simulink model "inverter"  (R2020a)
settings: Solver=VariableStepAuto  StartTime=0.0  StopTime=0.5  RelTol=1e-3
libraries: powerlib x15
settings Model: Creator=chrishao  LastModifiedBy=chrishao

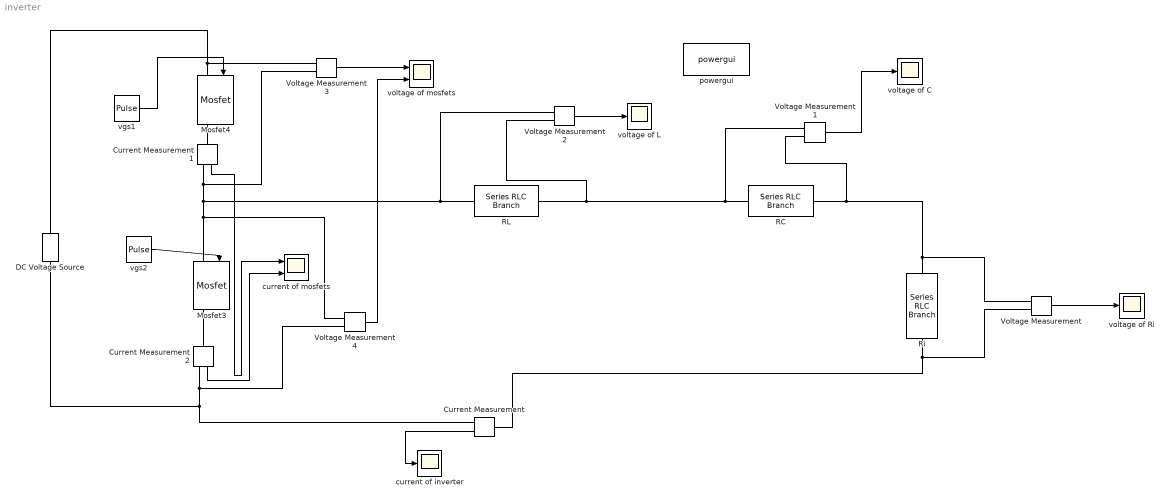
== system inverter ==
  Current Measurement : powerlib/Measurements/Current Measurement  PhasorSimulation=off  OutputType=Complex  PSBequivalent=0
  Current Measurement1 : powerlib/Measurements/Current Measurement  PhasorSimulation=off  OutputType=Complex  PSBequivalent=0
  Current Measurement2 : powerlib/Measurements/Current Measurement  PhasorSimulation=off  OutputType=Complex  PSBequivalent=0
  DC Voltage Source : powerlib/Electrical Sources/DC Voltage Source  Amplitude=180  Measurements=None
  Mosfet3 : powerlib/Power Electronics/Mosfet  Ron=1.4243  Lon=0  Rd=0.01  Vfd=0  IC=0  Rs=1e5  Cs=inf  Measurements=on
  Mosfet4 : powerlib/Power Electronics/Mosfet  Ron=1.4243  Lon=0  Rd=0.01  Vfd=0  IC=0  Rs=1e5  Cs=inf  Measurements=on
  RC : powerlib/Elements/Series RLC Branch  LConnTagsString=__new0  RConnTagsString=__new0  BranchType=RC  Resistance=0.7957  Inductance=675.2e-3  SetiL0=off  InitialCurrent=0  Capacitance=937.86e-12  Setx0=off  InitialVoltage=0  Measurements=None
  RL : powerlib/Elements/Series RLC Branch  LConnTagsString=__new0  RConnTagsString=__new0  BranchType=RL  Resistance=3.5090  Inductance=675.2e-6  SetiL0=off  InitialCurrent=0  Capacitance=1e-6  Setx0=off  InitialVoltage=0  Measurements=None
  Ri : powerlib/Elements/Series RLC Branch  LConnTagsString=__new0  RConnTagsString=__new0  BranchType=R  Resistance=137.4937  Inductance=675.2e-3  SetiL0=off  InitialCurrent=0  Capacitance=10e-9  Setx0=off  InitialVoltage=0  Measurements=None
  Voltage Measurement{,1..4} (5 alike) : powerlib/Measurements/Voltage Measurement  PhasorSimulation=off  OutputType=Complex  PSBequivalent=0
  current of inverter : Scope
  current of mosfets : Scope  NumInputPorts=2
  powergui : powerlib/powergui  Priority=1  SimulationMode=Continuous  SampleTime=50e-6  frequency=60  Iterations=50  frequencyindice=0  Pbase=100e6  ErrMax=1e-4  UnitsV=kV  UnitsW=MW  buscounter=0  FunctionMessages=off  echomessages=off  EnableUseOfTLC=off  CurrentSourceSwitches=off  DisableSnubberDevices=off  DisableRonSwitches=off  DisableVfSwitches=off  DisplayEquations=off  AutomaticDiscreteSolvers=off  SolverType=Tustin/Backward Euler (TBE)  Interpol=off  ExternalGateDelay=off  methode=off  Ts=100  x0status=blocks  SPID=on  SwTol=0  HookPort=off  NonlinearTolerance=1e-4  nMaxIteration=100  ContinueOnMaxIteration=off  RestoreLinks=warning  ResistiveCurrentMeasurement=off  Frange=[0:2:500]  Ylog=off  Xlog=on  ShowGrid=off  save=off  variable=ZData  structure=0  ZoomFFT=off  StartTime=0.0  cycles=1  DisplayStyle=1  fundamental=60  FreqAxis=off  MaxFrequency=1000  frequencyindicesteady=1  RmsSteady=1  display=off
  vgs1 : DiscretePulseGenerator  PulseType=Time based  Amplitude=15  Period=4.76e-6  PulseWidth=50
  vgs2 : DiscretePulseGenerator  PulseType=Time based  Amplitude=15  Period=4.76e-6  PulseWidth=50  PhaseDelay=2.38e-6
  voltage of C : Scope
  voltage of L : Scope
  voltage of Ri : Scope
  voltage of mosfets : Scope  NumInputPorts=2
  wires:
  vgs2/1 -> Mosfet3/1
  Current Measurement/1 -> current of inverter/1
  Voltage Measurement1/1 -> voltage of C/1
  Voltage Measurement2/1 -> voltage of L/1
  vgs1/1 -> Mosfet4/1
  Voltage Measurement/1 -> voltage of Ri/1
  Current Measurement2/1 -> current of mosfets/2
  Voltage Measurement3/1 -> voltage of mosfets/1
  Current Measurement1/1 -> current of mosfets/1
  Voltage Measurement4/1 -> voltage of mosfets/2
  connections:
  Ri/LConn1 -- RC/RConn1 -- Voltage Measurement1/LConn2 -- Voltage Measurement/LConn1
  Mosfet3/LConn1 -- Voltage Measurement4/LConn1 -- Voltage Measurement3/LConn2 -- Current Measurement1/RConn1 -- Voltage Measurement2/LConn1 -- RL/LConn1
  DC Voltage Source/RConn1 -- Voltage Measurement3/LConn1 -- Mosfet4/LConn1
  Current Measurement/LConn1 -- Ri/RConn1 -- Voltage Measurement/LConn2
  RC/LConn1 -- Voltage Measurement1/LConn1 -- RL/RConn1 -- Voltage Measurement2/LConn2
  DC Voltage Source/LConn1 -- Voltage Measurement4/LConn2 -- Current Measurement2/RConn1 -- Current Measurement/RConn1
  Current Measurement2/LConn1 -- Mosfet3/RConn1
  Mosfet4/RConn1 -- Current Measurement1/LConn1
